simulink model "SD_CIFB_3nd"  (R2016b)
settings: Solver=ode23t  StartTime=0.0  StopTime=L  FixedStep=1  RelTol=1e-6  AbsTol=1e-6
values from neighbouring files (symbols this model uses):
  a = amp(compt)    [QPSK.m]
  ai = amp(compt)    [Trace_RC.m]
  BW = fe/(2*OSR)    (= 0.0078125)    [Trace_RC.m]
  fin = fin_bin/Nfft    (= 0.00079345703125)    [DS_TB.m]    (also in Trace_RC.m)
  fircoeff = [1.60695392426680e-05 2.95841123026030e-05 5.48262790927617e-05 9.19832588239474e-05 0.000143686658983094 0.000212359882657570 0.000299965229015387 0.000407761225657029 0.000536071876123679 0.000684099631525166 0.000849796105711060 0.00102983168952252 0.00121960996869630 0.00141347333081234 0.00160490224533182 0.00178687182515771 0.00195224251942712 0.00209417001193910 0.00220655685058343 0.002284 ...(+463 chars)    [Trace_RC.m]
  fircoeff_fp = 0    [Trace_RC.m]
  fircoeff_round = round(fircoeff_round)    [Trace_RC.m]
undefined symbols (not defined in the file or in its folder): b, c, g
settings Model: ExtModeTrigMode=oneshot  ExtModeArmWhenConnect=off  ExtModeAutoUpdateStatusClock=off  Creator=sigma  LastModifiedBy=charles
settings DataIOCC: SaveFormat=Array  SignalLoggingSaveFormat=ModelDataLogs  SaveOutput=off  SaveTime=off  SignalLoggingName=sigsOut
settings OptimizationCC: BooleanDataType=off  ExpressionDepthLimit=2147483647  InitFltsAndDblsToZero=on  LifeSpan=inf
settings DebuggingCC: SaveWithParameterizedLinksMsg=none  UnderspecifiedInitializationDetection=Classic  MergeDetectMultiDrivingBlocksExec=none  SignalResolutionControl=TryResolveAllWithWarning  MultiTaskDSMMsg=warning  MultiTaskCondExecSysMsg=none  FcnCallInpInsideContextMsg=warning  StateNameClashWarn=warning  SFUnexpectedBacktrackingDiag=warning  SFNoUnconditionalDefaultTransitionDiag=warning  SFExecutionAtInitializationDiag=none
settings HardwareCC: ProdBitPerPointer=32  ProdBitPerSizeT=32  ProdBitPerPtrDiffT=32  ProdLargestAtomicFloat=None  ProdIntDivRoundTo=Undefined  ProdEndianess=Unspecified  ProdWordSize=32  ProdHWDeviceType=32-bit Generic  TargetUnknown=on
settings ModelReferenceCC: PropagateSignalLabelsOutOfModel=off
settings RTWCC: TemplateMakefile=grt_unix.tmf
settings GRTTargetCC: TargetLangStandard=C89/C90 (ANSI)  ModelReferenceCompliant=off  ParMdlRefBuildCompliant=off  CompOptLevelCompliant=off  ConcurrentExecutionCompliant=off  CombineOutputUpdateFcns=off  MatFileLogging=off  MATLABClassNameForMDSCustomization=Simulink.SoftwareTarget.TargetSpecificTriggerConfigurationBase  GRTInterface=on
settings ConfigComp: CovMetricSettings=dw  CovHtmlReporting=on  CovSaveCumulativeToWorkspaceVar=on  CovSaveSingleToWorkspaceVar=on  CovExternalEMLEnable=off

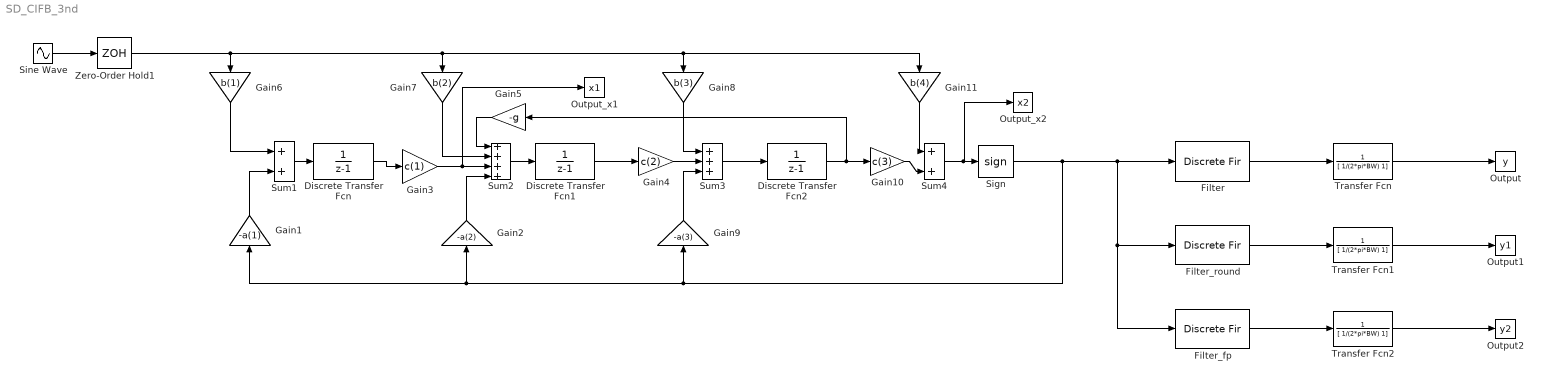
== system SD_CIFB_3nd ==
  Discrete Transfer Fcn : DiscreteTransferFcn  Denominator=[1 -1]
  Discrete Transfer Fcn1 : DiscreteTransferFcn  Denominator=[1 -1]
  Discrete Transfer Fcn2 : DiscreteTransferFcn  Denominator=[1 -1]
  "Filter " : DiscreteFir  Tag=BlockMethodSubSystem  Coefficients=fircoeff  InputProcessing=Columns as channels (frame based)
  "Filter_fp " : DiscreteFir  Tag=BlockMethodSubSystem  Coefficients=fircoeff_fp  InputProcessing=Columns as channels (frame based)
  Filter_round : DiscreteFir  Tag=BlockMethodSubSystem  Coefficients=fircoeff_round  InputProcessing=Columns as channels (frame based)
  Gain1 : Gain  Gain=-a(1)  SaturateOnIntegerOverflow=on  OutDataTypeStr=Inherit: Same as input  ParamDataTypeStr=Inherit: Same as input
  Gain10 : Gain  Gain=c(3)  SaturateOnIntegerOverflow=on  OutDataTypeStr=Inherit: Same as input  ParamDataTypeStr=Inherit: Same as input
  Gain11 : Gain  Gain=b(4)  SaturateOnIntegerOverflow=on  OutDataTypeStr=Inherit: Same as input  ParamDataTypeStr=Inherit: Same as input
  Gain2 : Gain  Gain=-a(2)  SaturateOnIntegerOverflow=on  OutDataTypeStr=Inherit: Same as input  ParamDataTypeStr=Inherit: Same as input
  Gain3 : Gain  Gain=c(1)  SaturateOnIntegerOverflow=on  OutDataTypeStr=Inherit: Same as input  ParamDataTypeStr=Inherit: Same as input
  Gain4 : Gain  Gain=c(2)  SaturateOnIntegerOverflow=on  OutDataTypeStr=Inherit: Same as input  ParamDataTypeStr=Inherit: Same as input
  Gain5 : Gain  Gain=-g  SaturateOnIntegerOverflow=on  OutDataTypeStr=Inherit: Same as input  ParamDataTypeStr=Inherit: Same as input
  Gain6 : Gain  Gain=b(1)  SaturateOnIntegerOverflow=on  OutDataTypeStr=Inherit: Same as input  ParamDataTypeStr=Inherit: Same as input
  Gain7 : Gain  Gain=b(2)  SaturateOnIntegerOverflow=on  OutDataTypeStr=Inherit: Same as input  ParamDataTypeStr=Inherit: Same as input
  Gain8 : Gain  Gain=b(3)  SaturateOnIntegerOverflow=on  OutDataTypeStr=Inherit: Same as input  ParamDataTypeStr=Inherit: Same as input
  Gain9 : Gain  Gain=-a(3)  SaturateOnIntegerOverflow=on  OutDataTypeStr=Inherit: Same as input  ParamDataTypeStr=Inherit: Same as input
  Output : ToWorkspace  VariableName=y  SampleTime=1
      settings: MaxDataPoints=N
  Output1 : ToWorkspace  VariableName=y1  SampleTime=1
      settings: MaxDataPoints=N
  Output2 : ToWorkspace  VariableName=y2  SampleTime=1
      settings: MaxDataPoints=N
  Output_x1 : ToWorkspace  VariableName=x1  SampleTime=1
      settings: MaxDataPoints=N
  Output_x2 : ToWorkspace  VariableName=x2  SampleTime=1
      settings: MaxDataPoints=N
  Sign : Signum
  Sine Wave : Sin  Amplitude=ai  Frequency=2*pi*fin  SampleTime=0
  Sum1 : Sum  SaturateOnIntegerOverflow=on  InputSameDT=on  OutDataTypeStr=Inherit: Same as first input
  Sum2 : Sum  Inputs=++++  SaturateOnIntegerOverflow=on  InputSameDT=on  OutDataTypeStr=Inherit: Same as first input
  Sum3 : Sum  Inputs=+++  SaturateOnIntegerOverflow=on  InputSameDT=on  OutDataTypeStr=Inherit: Same as first input
  Sum4 : Sum  SaturateOnIntegerOverflow=on  InputSameDT=on  OutDataTypeStr=Inherit: Same as first input
  Transfer Fcn : TransferFcn  Denominator=[ 1/(2*pi*BW) 1]
  Transfer Fcn1 : TransferFcn  Denominator=[ 1/(2*pi*BW) 1]
  Transfer Fcn2 : TransferFcn  Denominator=[ 1/(2*pi*BW) 1]
  Zero-Order Hold1 : ZeroOrderHold
  wires:
  Gain1/1 -> Sum1/2
  Sine Wave/1 -> Zero-Order Hold1/1
  Gain2/1 -> Sum2/4
  Discrete Transfer Fcn/1 -> Gain3/1
  Sum1/1 -> Discrete Transfer Fcn/1
  Gain3/1 -> Sum2/3, Output_x1/1
  Sum2/1 -> Discrete Transfer Fcn1/1
  Discrete Transfer Fcn1/1 -> Gain4/1
  Gain6/1 -> Sum1/1
  Zero-Order Hold1/1 -> Gain11/1, Gain8/1, Gain7/1, Gain6/1
  Gain7/1 -> Sum2/2
  Gain4/1 -> Sum3/2
  Gain8/1 -> Sum3/1
  Gain5/1 -> Sum2/1
  Gain9/1 -> Sum3/3
  Discrete Transfer Fcn2/1 -> Gain5/1, Gain10/1
  Sum3/1 -> Discrete Transfer Fcn2/1
  Gain10/1 -> Sum4/2
  Sum4/1 -> Output_x2/1, Sign/1
  Gain11/1 -> Sum4/1
  Sign/1 -> "Filter_fp "/1, Filter_round/1, "Filter "/1, Gain9/1, Gain1/1, Gain2/1
  "Filter "/1 -> Transfer Fcn/1
  Filter_round/1 -> Transfer Fcn1/1
  "Filter_fp "/1 -> Transfer Fcn2/1
  Transfer Fcn2/1 -> Output2/1
  Transfer Fcn/1 -> Output/1
  Transfer Fcn1/1 -> Output1/1
